simulink model "humanTestController"  (Simulink 9.1)
settings: Solver=FixedStepDiscrete  StartTime=0.0  StopTime=inf  FixedStep=Config.Ts  RelTol=1e-3  EnableMultiTasking=on
InitFcn:
  | initHumanController
values from neighbouring files (symbols this model uses):
  HUMAN_ON_GAZEBO = true    [initHumanController.m]
libraries: WBToolboxLibrary x17
settings Model: SuppressorTable=22 serialization::archive 11 0 6 0 0 0 1 0  Creator=yeshi  LastModifiedBy=yeshi
settings DataIOCC: SaveFormat=Dataset
settings DebuggingCC: UnderspecifiedInitializationDetection=Simplified  MergeDetectMultiDrivingBlocksExec=error
settings HardwareCC: ProdBitPerPointer=64  ProdBitPerSizeT=64  ProdBitPerPtrDiffT=64  ProdLargestAtomicFloat=Float  ProdIntDivRoundTo=Zero  ProdEndianess=LittleEndian  ProdWordSize=64  ProdHWDeviceType=Intel->x86-64 (Windows64)
settings ModelReferenceCC: PropagateSignalLabelsOutOfModel=on
settings GRTTargetCC: GeneratePreprocessorConditionals=Disable all  CombineOutputUpdateFcns=on  GRTInterface=off

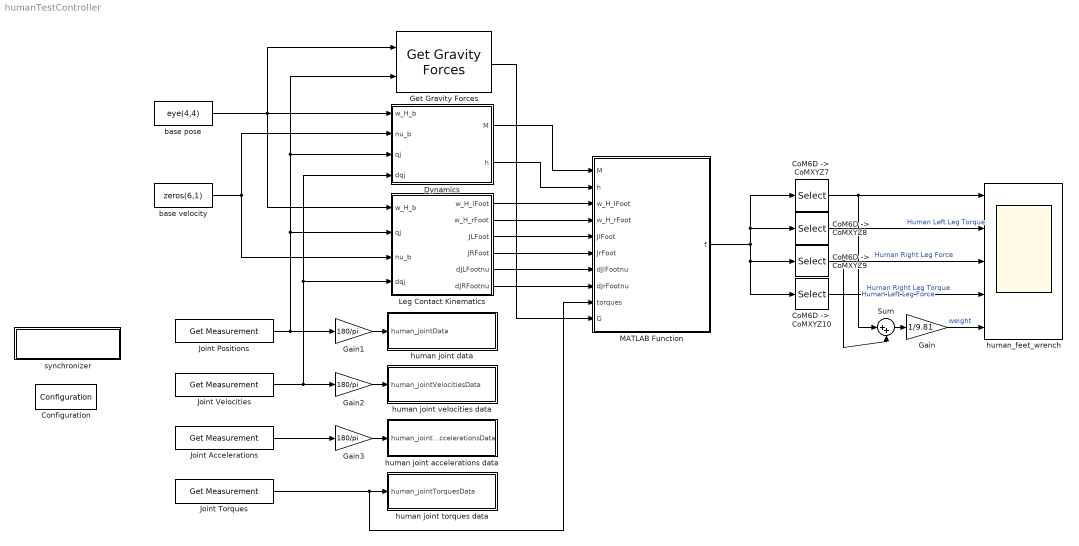
== system humanTestController ==
  "CoM6D ->  CoMXYZ10" : Selector  InputPortWidth=12  IndexOptions=Index vector (dialog)  Indices=[10 11 12]  OutputSizes=1
  "CoM6D ->  CoMXYZ7" : Selector  InputPortWidth=12  IndexOptions=Index vector (dialog)  Indices=[1 2 3]  OutputSizes=1
  "CoM6D ->  CoMXYZ8" : Selector  InputPortWidth=12  IndexOptions=Index vector (dialog)  Indices=[4 5 6]  OutputSizes=1
  "CoM6D ->  CoMXYZ9" : Selector  InputPortWidth=12  IndexOptions=Index vector (dialog)  Indices=[7 8 9]  OutputSizes=1
  Configuration : WBToolboxLibrary/Utilities/Configuration  ConfigSource=Workspace  ConfigObject='HUMAN.WBTConfigRobot'
      settings: SourceProductName=Whole Body Toolbox
  Dynamics : Subsystem
  Gain : Gain  Gain=1/9.81
  Gain1 : Gain  Gain=180/pi
  Gain2 : Gain  Gain=180/pi
  Gain3 : Gain  Gain=180/pi
  Get Gravity Forces : WBToolboxLibrary/wholeBodyModel/Dynamics/Get Gravity Forces
      settings: SourceProductName=Whole Body Toolbox
  Joint Accelerations : WBToolboxLibrary/wholeBodyStates/Get Measurement  measuredType=Joints Acceleration
      settings: SourceProductName=Whole Body Toolbox
  Joint Positions : WBToolboxLibrary/wholeBodyStates/Get Measurement  measuredType=Joints Position
      settings: SourceProductName=Whole Body Toolbox
  Joint Torques : WBToolboxLibrary/wholeBodyStates/Get Measurement  measuredType=Joints Torque
      settings: SourceProductName=Whole Body Toolbox
  Joint Velocities : WBToolboxLibrary/wholeBodyStates/Get Measurement  measuredType=Joints Velocity
      settings: SourceProductName=Whole Body Toolbox
  Leg Contact Kinematics : Subsystem
  MATLAB Function : MATLAB Function  TreatAsAtomicUnit=on
  Sum : Sum  Inputs=|++
  base pose : Constant  Value=eye(4,4)
  base velocity : Constant  Value=zeros(6,1)
  human joint accelerations data : Subsystem
  human joint data : Subsystem
  human joint torques data : Subsystem
  human joint velocities data : Subsystem
  human_feet_wrench : Scope  NumInputPorts=5
  synchronizer : Subsystem
      mask Display: disp('SYNCHRONIZER')
  wires:
  Joint Positions/1 -> Leg Contact Kinematics/2(qj), Dynamics/3(qj), Get Gravity Forces/2, Gain1/1
  Gain2/1 -> human joint velocities data/1(human_jointVelocitiesData)
  Gain3/1 -> human joint accelerations data/1(human_jointAccelerationsData)
  Joint Velocities/1 -> Leg Contact Kinematics/4(dqj), Dynamics/4(dqj), Gain2/1
  Joint Accelerations/1 -> Gain3/1
  Joint Torques/1 -> MATLAB Function/9(torques), human joint torques data/1(human_jointTorquesData)
  base pose/1 -> Dynamics/1(w_H_b), Get Gravity Forces/1, Leg Contact Kinematics/1(w_H_b)
  base velocity/1 -> Leg Contact Kinematics/3(nu_b), Dynamics/2(nu_b)
  Gain1/1 -> human joint data/1(human_jointData)
  Leg Contact Kinematics/1(w_H_lFoot) -> MATLAB Function/3(w_H_lFoot)
  Leg Contact Kinematics/2(w_H_rFoot) -> MATLAB Function/4(w_H_rFoot)
  Leg Contact Kinematics/3(JLFoot) -> MATLAB Function/5(JlFoot)
  Leg Contact Kinematics/4(JRFoot) -> MATLAB Function/6(JrFoot)
  Leg Contact Kinematics/5(dJLFootnu) -> MATLAB Function/7(dJlFootnu)
  Leg Contact Kinematics/6(dJRFootnu) -> MATLAB Function/8(dJrFootnu)
  Dynamics/2(h) -> MATLAB Function/2(h)
  Dynamics/1(M) -> MATLAB Function/1(M)
  "CoM6D ->  CoMXYZ8"/1 -> human_feet_wrench/2  "Human Left Leg Torque"
  MATLAB Function/1(f) -> "CoM6D ->  CoMXYZ10"/1, "CoM6D ->  CoMXYZ9"/1, "CoM6D ->  CoMXYZ8"/1, "CoM6D ->  CoMXYZ7"/1
  "CoM6D ->  CoMXYZ10"/1 -> human_feet_wrench/4  "Human Right Leg Torque"
  "CoM6D ->  CoMXYZ7"/1 -> Sum/1, human_feet_wrench/1  "Human Left Leg Force"
  "CoM6D ->  CoMXYZ9"/1 -> Sum/2, human_feet_wrench/3  "Human Right Leg Force"
  Get Gravity Forces/1 -> MATLAB Function/10(G)
  Sum/1 -> Gain/1
  Gain/1 -> human_feet_wrench/5  "weight"

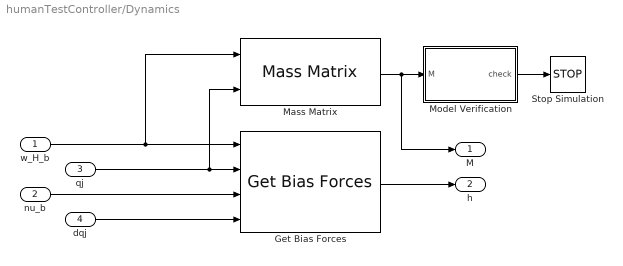
== system humanTestController/Dynamics ==
  w_H_b : Inport
  nu_b : Inport  Port=2
  qj : Inport  Port=3
  dqj : Inport  Port=4
  Get Bias Forces : WBToolboxLibrary/wholeBodyModel/Dynamics/Get Bias Forces
      settings: SourceProductName=Whole Body Toolbox
  Mass Matrix : WBToolboxLibrary/wholeBodyModel/Dynamics/Mass Matrix
      settings: SourceProductName=Whole Body Toolbox
  Model Verification : MATLAB Function  TreatAsAtomicUnit=on
  Stop Simulation : Stop
  M : Outport
  h : Outport  Port=2
  wires:
  dqj/1 -> Get Bias Forces/4
  w_H_b/1 -> Get Bias Forces/1, Mass Matrix/1
  qj/1 -> Get Bias Forces/2, Mass Matrix/2
  Mass Matrix/1 -> M/1, Model Verification/1(M)
  nu_b/1 -> Get Bias Forces/3
  Get Bias Forces/1 -> h/1
  Model Verification/1(check) -> Stop Simulation/1

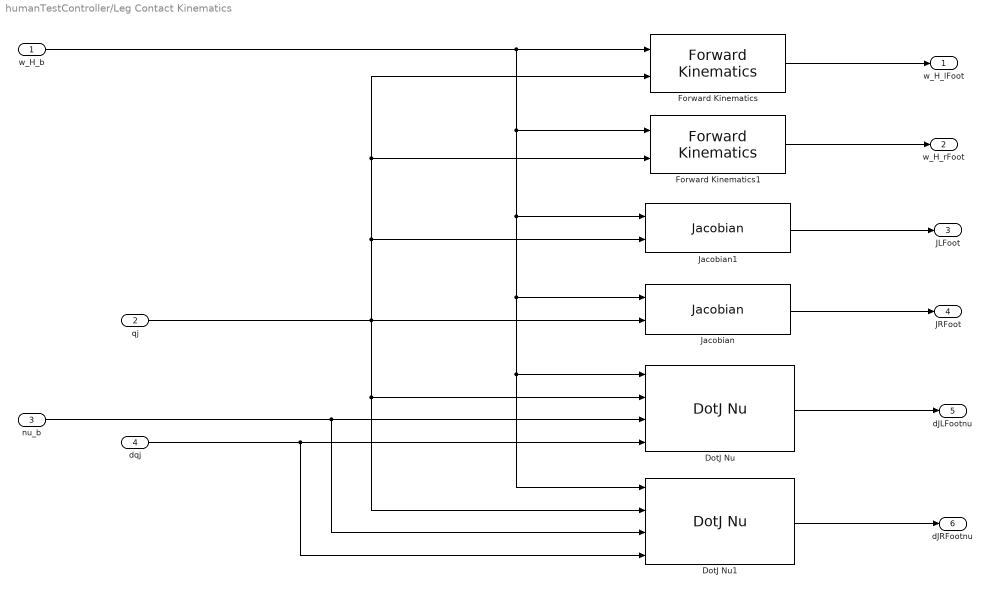
== system humanTestController/Leg Contact Kinematics ==
  w_H_b : Inport
  qj : Inport  Port=2
  nu_b : Inport  Port=3
  dqj : Inport  Port=4
  DotJ Nu : WBToolboxLibrary/wholeBodyModel/Jacobians/DotJ Nu  frameName=HUMAN_Frames.LEFT_FOOT
      settings: SourceProductName=Whole Body Toolbox
  DotJ Nu1 : WBToolboxLibrary/wholeBodyModel/Jacobians/DotJ Nu  frameName=HUMAN_Frames.RIGHT_FOOT
      settings: SourceProductName=Whole Body Toolbox
  Forward Kinematics : WBToolboxLibrary/wholeBodyModel/Kinematics/Forward Kinematics  frameName=HUMAN_Frames.LEFT_FOOT
      settings: SourceProductName=Whole Body Toolbox
  Forward Kinematics1 : WBToolboxLibrary/wholeBodyModel/Kinematics/Forward Kinematics  frameName=HUMAN_Frames.RIGHT_FOOT
      settings: SourceProductName=Whole Body Toolbox
  Jacobian : WBToolboxLibrary/wholeBodyModel/Jacobians/Jacobian  frameName=HUMAN_Frames.RIGHT_FOOT
      settings: SourceProductName=Whole Body Toolbox
  Jacobian1 : WBToolboxLibrary/wholeBodyModel/Jacobians/Jacobian  frameName=HUMAN_Frames.LEFT_FOOT
      settings: SourceProductName=Whole Body Toolbox
  w_H_lFoot : Outport
  w_H_rFoot : Outport  Port=2
  JLFoot : Outport  Port=3
  JRFoot : Outport  Port=4
  dJLFootnu : Outport  Port=5
  dJRFootnu : Outport  Port=6
  wires:
  DotJ Nu/1 -> dJLFootnu/1
  DotJ Nu1/1 -> dJRFootnu/1
  Jacobian/1 -> JRFoot/1
  Forward Kinematics1/1 -> w_H_rFoot/1
  nu_b/1 -> DotJ Nu1/3, DotJ Nu/3
  qj/1 -> Forward Kinematics/2, Forward Kinematics1/2, Jacobian1/2, Jacobian/2, DotJ Nu/2, DotJ Nu1/2
  w_H_b/1 -> Forward Kinematics1/1, Jacobian1/1, DotJ Nu/1, DotJ Nu1/1, Jacobian/1, Forward Kinematics/1
  dqj/1 -> DotJ Nu1/4, DotJ Nu/4
  Jacobian1/1 -> JLFoot/1
  Forward Kinematics/1 -> w_H_lFoot/1

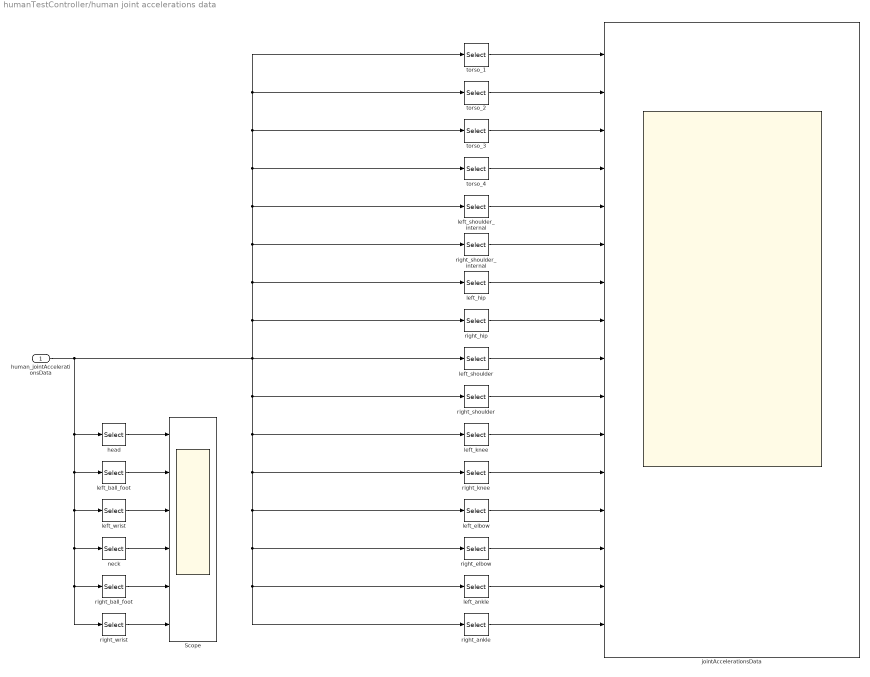
== system humanTestController/human joint accelerations data ==
  human_jointAccelerationsData : Inport
  Scope : Scope  NumInputPorts=6
  head : Selector  InputPortWidth=66  IndexOptions=Index vector (dialog)  Indices=[16 17 18]  OutputSizes=1
  jointAccelerationsData : Scope  NumInputPorts=16
  left_ankle : Selector  InputPortWidth=66  IndexOptions=Index vector (dialog)  Indices=[61 62 63]  OutputSizes=1
  left_ball_foot : Selector  InputPortWidth=66  IndexOptions=Index vector (dialog)  Indices=[64 65 66]  OutputSizes=1
  left_elbow : Selector  InputPortWidth=66  IndexOptions=Index vector (dialog)  Indices=[37 38 39]  OutputSizes=1
  left_hip : Selector  InputPortWidth=66  IndexOptions=Index vector (dialog)  Indices=[55 56 57]  OutputSizes=1
  left_knee : Selector  InputPortWidth=66  IndexOptions=Index vector (dialog)  Indices=[58 59 60]  OutputSizes=1
  left_shoulder : Selector  InputPortWidth=66  IndexOptions=Index vector (dialog)  Indices=[34 35 36]  OutputSizes=1
  left_shoulder_internal : Selector  InputPortWidth=66  IndexOptions=Index vector (dialog)  Indices=[31 32 33]  OutputSizes=1
  left_wrist : Selector  InputPortWidth=66  IndexOptions=Index vector (dialog)  Indices=[40 41 42]  OutputSizes=1
  neck : Selector  InputPortWidth=66  IndexOptions=Index vector (dialog)  Indices=[13 14 15]  OutputSizes=1
  right_ankle : Selector  InputPortWidth=66  IndexOptions=Index vector (dialog)  Indices=[49 50 51]  OutputSizes=1
  right_ball_foot : Selector  InputPortWidth=66  IndexOptions=Index vector (dialog)  Indices=[52 53 54]  OutputSizes=1
  right_elbow : Selector  InputPortWidth=66  IndexOptions=Index vector (dialog)  Indices=[25 26 27]  OutputSizes=1
  right_hip : Selector  InputPortWidth=66  IndexOptions=Index vector (dialog)  Indices=[43 44 45]  OutputSizes=1
  right_knee : Selector  InputPortWidth=66  IndexOptions=Index vector (dialog)  Indices=[46 47 48]  OutputSizes=1
  right_shoulder : Selector  InputPortWidth=66  IndexOptions=Index vector (dialog)  Indices=[22 23 24]  OutputSizes=1
  right_shoulder_internal : Selector  InputPortWidth=66  IndexOptions=Index vector (dialog)  Indices=[19 20 21]  OutputSizes=1
  right_wrist : Selector  InputPortWidth=66  IndexOptions=Index vector (dialog)  Indices=[28 29 30]  OutputSizes=1
  torso_1 : Selector  InputPortWidth=66  IndexOptions=Index vector (dialog)  Indices=[10 11 12]  OutputSizes=1
  torso_2 : Selector  InputPortWidth=66  IndexOptions=Index vector (dialog)  Indices=[7 8 9]  OutputSizes=1
  torso_3 : Selector  InputPortWidth=66  IndexOptions=Index vector (dialog)  Indices=[4 5 6]  OutputSizes=1
  torso_4 : Selector  InputPortWidth=66  IndexOptions=Index vector (dialog)  Indices=[1 2 3]  OutputSizes=1
  wires:
  torso_1/1 -> jointAccelerationsData/1
  torso_4/1 -> jointAccelerationsData/4
  torso_3/1 -> jointAccelerationsData/3
  torso_2/1 -> jointAccelerationsData/2
  right_shoulder_internal/1 -> jointAccelerationsData/6
  left_shoulder_internal/1 -> jointAccelerationsData/5
  left_hip/1 -> jointAccelerationsData/7
  right_hip/1 -> jointAccelerationsData/8
  left_shoulder/1 -> jointAccelerationsData/9
  right_shoulder/1 -> jointAccelerationsData/10
  left_knee/1 -> jointAccelerationsData/11
  right_knee/1 -> jointAccelerationsData/12
  left_elbow/1 -> jointAccelerationsData/13
  right_elbow/1 -> jointAccelerationsData/14
  left_ankle/1 -> jointAccelerationsData/15
  right_ankle/1 -> jointAccelerationsData/16
  human_jointAccelerationsData/1 -> head/1, left_ball_foot/1, left_wrist/1, neck/1, right_ball_foot/1, right_wrist/1, left_shoulder/1, right_hip/1, left_hip/1, right_shoulder_internal/1, torso_1/1, torso_2/1, torso_3/1, torso_4/1, left_shoulder_internal/1, right_shoulder/1, left_knee/1, right_knee/1, left_elbow/1, right_elbow/1, right_ankle/1, left_ankle/1
  head/1 -> Scope/1
  left_ball_foot/1 -> Scope/2
  left_wrist/1 -> Scope/3
  neck/1 -> Scope/4
  right_ball_foot/1 -> Scope/5
  right_wrist/1 -> Scope/6

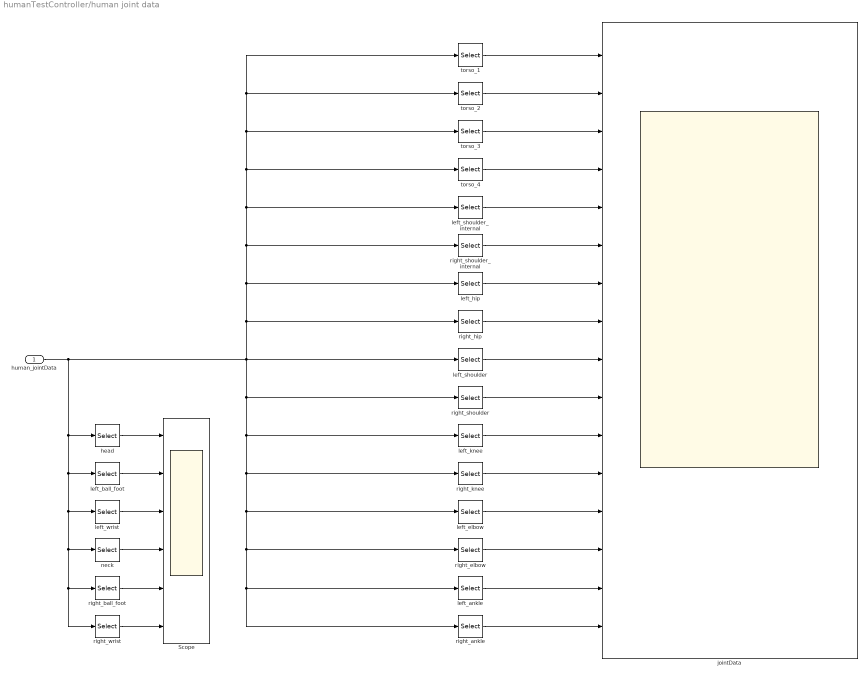
== system humanTestController/human joint data ==
  human_jointData : Inport
  Scope : Scope  NumInputPorts=6
  head : Selector  InputPortWidth=66  IndexOptions=Index vector (dialog)  Indices=[16 17 18]  OutputSizes=1
  jointData : Scope  NumInputPorts=16
  left_ankle : Selector  InputPortWidth=66  IndexOptions=Index vector (dialog)  Indices=[61 62 63]  OutputSizes=1
  left_ball_foot : Selector  InputPortWidth=66  IndexOptions=Index vector (dialog)  Indices=[64 65 66]  OutputSizes=1
  left_elbow : Selector  InputPortWidth=66  IndexOptions=Index vector (dialog)  Indices=[37 38 39]  OutputSizes=1
  left_hip : Selector  InputPortWidth=66  IndexOptions=Index vector (dialog)  Indices=[55 56 57]  OutputSizes=1
  left_knee : Selector  InputPortWidth=66  IndexOptions=Index vector (dialog)  Indices=[58 59 60]  OutputSizes=1
  left_shoulder : Selector  InputPortWidth=66  IndexOptions=Index vector (dialog)  Indices=[34 35 36]  OutputSizes=1
  left_shoulder_internal : Selector  InputPortWidth=66  IndexOptions=Index vector (dialog)  Indices=[31 32 33]  OutputSizes=1
  left_wrist : Selector  InputPortWidth=66  IndexOptions=Index vector (dialog)  Indices=[40 41 42]  OutputSizes=1
  neck : Selector  InputPortWidth=66  IndexOptions=Index vector (dialog)  Indices=[13 14 15]  OutputSizes=1
  right_ankle : Selector  InputPortWidth=66  IndexOptions=Index vector (dialog)  Indices=[49 50 51]  OutputSizes=1
  right_ball_foot : Selector  InputPortWidth=66  IndexOptions=Index vector (dialog)  Indices=[52 53 54]  OutputSizes=1
  right_elbow : Selector  InputPortWidth=66  IndexOptions=Index vector (dialog)  Indices=[25 26 27]  OutputSizes=1
  right_hip : Selector  InputPortWidth=66  IndexOptions=Index vector (dialog)  Indices=[43 44 45]  OutputSizes=1
  right_knee : Selector  InputPortWidth=66  IndexOptions=Index vector (dialog)  Indices=[46 47 48]  OutputSizes=1
  right_shoulder : Selector  InputPortWidth=66  IndexOptions=Index vector (dialog)  Indices=[22 23 24]  OutputSizes=1
  right_shoulder_internal : Selector  InputPortWidth=66  IndexOptions=Index vector (dialog)  Indices=[19 20 21]  OutputSizes=1
  right_wrist : Selector  InputPortWidth=66  IndexOptions=Index vector (dialog)  Indices=[28 29 30]  OutputSizes=1
  torso_1 : Selector  InputPortWidth=66  IndexOptions=Index vector (dialog)  Indices=[10 11 12]  OutputSizes=1
  torso_2 : Selector  InputPortWidth=66  IndexOptions=Index vector (dialog)  Indices=[7 8 9]  OutputSizes=1
  torso_3 : Selector  InputPortWidth=66  IndexOptions=Index vector (dialog)  Indices=[4 5 6]  OutputSizes=1
  torso_4 : Selector  InputPortWidth=66  IndexOptions=Index vector (dialog)  Indices=[1 2 3]  OutputSizes=1
  wires:
  torso_1/1 -> jointData/1
  torso_4/1 -> jointData/4
  torso_3/1 -> jointData/3
  torso_2/1 -> jointData/2
  right_shoulder_internal/1 -> jointData/6
  left_shoulder_internal/1 -> jointData/5
  left_hip/1 -> jointData/7
  right_hip/1 -> jointData/8
  left_shoulder/1 -> jointData/9
  right_shoulder/1 -> jointData/10
  left_knee/1 -> jointData/11
  right_knee/1 -> jointData/12
  left_elbow/1 -> jointData/13
  right_elbow/1 -> jointData/14
  left_ankle/1 -> jointData/15
  right_ankle/1 -> jointData/16
  human_jointData/1 -> head/1, left_ball_foot/1, left_wrist/1, neck/1, right_ball_foot/1, right_wrist/1, left_shoulder/1, right_hip/1, left_hip/1, right_shoulder_internal/1, torso_1/1, torso_2/1, torso_3/1, torso_4/1, left_shoulder_internal/1, right_shoulder/1, left_knee/1, right_knee/1, left_elbow/1, right_elbow/1, right_ankle/1, left_ankle/1
  head/1 -> Scope/1
  left_ball_foot/1 -> Scope/2
  left_wrist/1 -> Scope/3
  neck/1 -> Scope/4
  right_ball_foot/1 -> Scope/5
  right_wrist/1 -> Scope/6

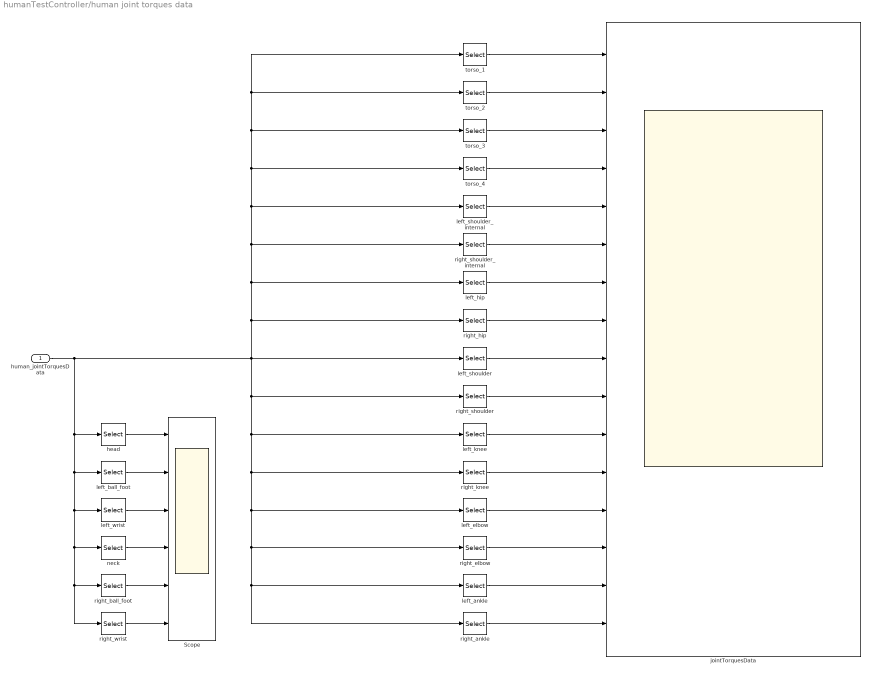
== system humanTestController/human joint torques data ==
  human_jointTorquesData : Inport
  Scope : Scope  NumInputPorts=6
  head : Selector  InputPortWidth=66  IndexOptions=Index vector (dialog)  Indices=[16 17 18]  OutputSizes=1
  jointTorquesData : Scope  NumInputPorts=16
  left_ankle : Selector  InputPortWidth=66  IndexOptions=Index vector (dialog)  Indices=[61 62 63]  OutputSizes=1
  left_ball_foot : Selector  InputPortWidth=66  IndexOptions=Index vector (dialog)  Indices=[64 65 66]  OutputSizes=1
  left_elbow : Selector  InputPortWidth=66  IndexOptions=Index vector (dialog)  Indices=[37 38 39]  OutputSizes=1
  left_hip : Selector  InputPortWidth=66  IndexOptions=Index vector (dialog)  Indices=[55 56 57]  OutputSizes=1
  left_knee : Selector  InputPortWidth=66  IndexOptions=Index vector (dialog)  Indices=[58 59 60]  OutputSizes=1
  left_shoulder : Selector  InputPortWidth=66  IndexOptions=Index vector (dialog)  Indices=[34 35 36]  OutputSizes=1
  left_shoulder_internal : Selector  InputPortWidth=66  IndexOptions=Index vector (dialog)  Indices=[31 32 33]  OutputSizes=1
  left_wrist : Selector  InputPortWidth=66  IndexOptions=Index vector (dialog)  Indices=[40 41 42]  OutputSizes=1
  neck : Selector  InputPortWidth=66  IndexOptions=Index vector (dialog)  Indices=[13 14 15]  OutputSizes=1
  right_ankle : Selector  InputPortWidth=66  IndexOptions=Index vector (dialog)  Indices=[49 50 51]  OutputSizes=1
  right_ball_foot : Selector  InputPortWidth=66  IndexOptions=Index vector (dialog)  Indices=[52 53 54]  OutputSizes=1
  right_elbow : Selector  InputPortWidth=66  IndexOptions=Index vector (dialog)  Indices=[25 26 27]  OutputSizes=1
  right_hip : Selector  InputPortWidth=66  IndexOptions=Index vector (dialog)  Indices=[43 44 45]  OutputSizes=1
  right_knee : Selector  InputPortWidth=66  IndexOptions=Index vector (dialog)  Indices=[46 47 48]  OutputSizes=1
  right_shoulder : Selector  InputPortWidth=66  IndexOptions=Index vector (dialog)  Indices=[22 23 24]  OutputSizes=1
  right_shoulder_internal : Selector  InputPortWidth=66  IndexOptions=Index vector (dialog)  Indices=[19 20 21]  OutputSizes=1
  right_wrist : Selector  InputPortWidth=66  IndexOptions=Index vector (dialog)  Indices=[28 29 30]  OutputSizes=1
  torso_1 : Selector  InputPortWidth=66  IndexOptions=Index vector (dialog)  Indices=[10 11 12]  OutputSizes=1
  torso_2 : Selector  InputPortWidth=66  IndexOptions=Index vector (dialog)  Indices=[7 8 9]  OutputSizes=1
  torso_3 : Selector  InputPortWidth=66  IndexOptions=Index vector (dialog)  Indices=[4 5 6]  OutputSizes=1
  torso_4 : Selector  InputPortWidth=66  IndexOptions=Index vector (dialog)  Indices=[1 2 3]  OutputSizes=1
  wires:
  torso_1/1 -> jointTorquesData/1
  torso_4/1 -> jointTorquesData/4
  torso_3/1 -> jointTorquesData/3
  torso_2/1 -> jointTorquesData/2
  right_shoulder_internal/1 -> jointTorquesData/6
  left_shoulder_internal/1 -> jointTorquesData/5
  left_hip/1 -> jointTorquesData/7
  right_hip/1 -> jointTorquesData/8
  left_shoulder/1 -> jointTorquesData/9
  right_shoulder/1 -> jointTorquesData/10
  left_knee/1 -> jointTorquesData/11
  right_knee/1 -> jointTorquesData/12
  left_elbow/1 -> jointTorquesData/13
  right_elbow/1 -> jointTorquesData/14
  left_ankle/1 -> jointTorquesData/15
  right_ankle/1 -> jointTorquesData/16
  human_jointTorquesData/1 -> head/1, left_ball_foot/1, left_wrist/1, neck/1, right_ball_foot/1, right_wrist/1, left_shoulder/1, right_hip/1, left_hip/1, right_shoulder_internal/1, torso_1/1, torso_2/1, torso_3/1, torso_4/1, left_shoulder_internal/1, right_shoulder/1, left_knee/1, right_knee/1, left_elbow/1, right_elbow/1, right_ankle/1, left_ankle/1
  head/1 -> Scope/1
  left_ball_foot/1 -> Scope/2
  left_wrist/1 -> Scope/3
  neck/1 -> Scope/4
  right_ball_foot/1 -> Scope/5
  right_wrist/1 -> Scope/6

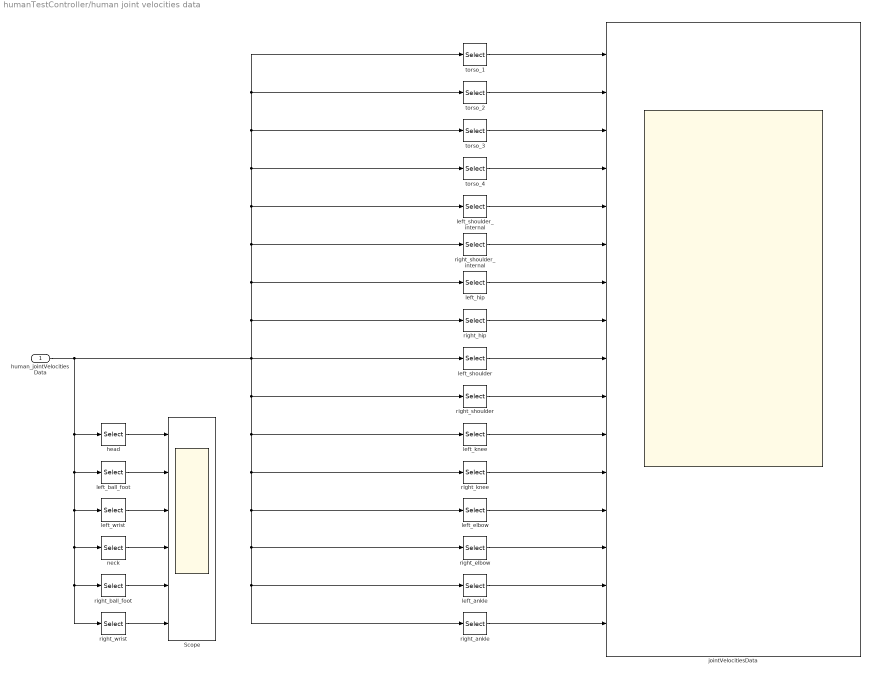
== system humanTestController/human joint velocities data ==
  human_jointVelocitiesData : Inport
  Scope : Scope  NumInputPorts=6
  head : Selector  InputPortWidth=66  IndexOptions=Index vector (dialog)  Indices=[16 17 18]  OutputSizes=1
  jointVelocitiesData : Scope  NumInputPorts=16
  left_ankle : Selector  InputPortWidth=66  IndexOptions=Index vector (dialog)  Indices=[61 62 63]  OutputSizes=1
  left_ball_foot : Selector  InputPortWidth=66  IndexOptions=Index vector (dialog)  Indices=[64 65 66]  OutputSizes=1
  left_elbow : Selector  InputPortWidth=66  IndexOptions=Index vector (dialog)  Indices=[37 38 39]  OutputSizes=1
  left_hip : Selector  InputPortWidth=66  IndexOptions=Index vector (dialog)  Indices=[55 56 57]  OutputSizes=1
  left_knee : Selector  InputPortWidth=66  IndexOptions=Index vector (dialog)  Indices=[58 59 60]  OutputSizes=1
  left_shoulder : Selector  InputPortWidth=66  IndexOptions=Index vector (dialog)  Indices=[34 35 36]  OutputSizes=1
  left_shoulder_internal : Selector  InputPortWidth=66  IndexOptions=Index vector (dialog)  Indices=[31 32 33]  OutputSizes=1
  left_wrist : Selector  InputPortWidth=66  IndexOptions=Index vector (dialog)  Indices=[40 41 42]  OutputSizes=1
  neck : Selector  InputPortWidth=66  IndexOptions=Index vector (dialog)  Indices=[13 14 15]  OutputSizes=1
  right_ankle : Selector  InputPortWidth=66  IndexOptions=Index vector (dialog)  Indices=[49 50 51]  OutputSizes=1
  right_ball_foot : Selector  InputPortWidth=66  IndexOptions=Index vector (dialog)  Indices=[52 53 54]  OutputSizes=1
  right_elbow : Selector  InputPortWidth=66  IndexOptions=Index vector (dialog)  Indices=[25 26 27]  OutputSizes=1
  right_hip : Selector  InputPortWidth=66  IndexOptions=Index vector (dialog)  Indices=[43 44 45]  OutputSizes=1
  right_knee : Selector  InputPortWidth=66  IndexOptions=Index vector (dialog)  Indices=[46 47 48]  OutputSizes=1
  right_shoulder : Selector  InputPortWidth=66  IndexOptions=Index vector (dialog)  Indices=[22 23 24]  OutputSizes=1
  right_shoulder_internal : Selector  InputPortWidth=66  IndexOptions=Index vector (dialog)  Indices=[19 20 21]  OutputSizes=1
  right_wrist : Selector  InputPortWidth=66  IndexOptions=Index vector (dialog)  Indices=[28 29 30]  OutputSizes=1
  torso_1 : Selector  InputPortWidth=66  IndexOptions=Index vector (dialog)  Indices=[10 11 12]  OutputSizes=1
  torso_2 : Selector  InputPortWidth=66  IndexOptions=Index vector (dialog)  Indices=[7 8 9]  OutputSizes=1
  torso_3 : Selector  InputPortWidth=66  IndexOptions=Index vector (dialog)  Indices=[4 5 6]  OutputSizes=1
  torso_4 : Selector  InputPortWidth=66  IndexOptions=Index vector (dialog)  Indices=[1 2 3]  OutputSizes=1
  wires:
  torso_1/1 -> jointVelocitiesData/1
  torso_4/1 -> jointVelocitiesData/4
  torso_3/1 -> jointVelocitiesData/3
  torso_2/1 -> jointVelocitiesData/2
  right_shoulder_internal/1 -> jointVelocitiesData/6
  left_shoulder_internal/1 -> jointVelocitiesData/5
  left_hip/1 -> jointVelocitiesData/7
  right_hip/1 -> jointVelocitiesData/8
  left_shoulder/1 -> jointVelocitiesData/9
  right_shoulder/1 -> jointVelocitiesData/10
  left_knee/1 -> jointVelocitiesData/11
  right_knee/1 -> jointVelocitiesData/12
  left_elbow/1 -> jointVelocitiesData/13
  right_elbow/1 -> jointVelocitiesData/14
  left_ankle/1 -> jointVelocitiesData/15
  right_ankle/1 -> jointVelocitiesData/16
  human_jointVelocitiesData/1 -> head/1, left_ball_foot/1, left_wrist/1, neck/1, right_ball_foot/1, right_wrist/1, left_shoulder/1, right_hip/1, left_hip/1, right_shoulder_internal/1, torso_1/1, torso_2/1, torso_3/1, torso_4/1, left_shoulder_internal/1, right_shoulder/1, left_knee/1, right_knee/1, left_elbow/1, right_elbow/1, right_ankle/1, left_ankle/1
  head/1 -> Scope/1
  left_ball_foot/1 -> Scope/2
  left_wrist/1 -> Scope/3
  neck/1 -> Scope/4
  right_ball_foot/1 -> Scope/5
  right_wrist/1 -> Scope/6

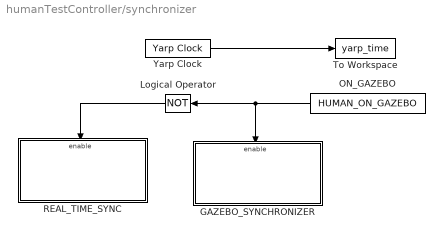
== system humanTestController/synchronizer ==
  GAZEBO_SYNCHRONIZER : Subsystem
  Logical Operator : Logic  Operator=NOT  AllPortsSameDT=off  OutDataTypeStr=boolean
  "ON_GAZEBO " : Constant  Value=HUMAN_ON_GAZEBO
  REAL_TIME_SYNC : Subsystem
  To Workspace : ToWorkspace  VariableName=yarp_time  SaveFormat=Structure With Time  SampleTime=-1
  Yarp Clock : WBToolboxLibrary/Utilities/Yarp Clock
      settings: SourceProductName=Whole Body Toolbox
  wires:
  Logical Operator/1 -> REAL_TIME_SYNC/Enable
  "ON_GAZEBO "/1 -> GAZEBO_SYNCHRONIZER/Enable, Logical Operator/1
  Yarp Clock/1 -> To Workspace/1

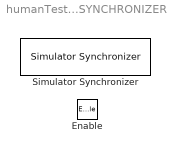
== system humanTestController/synchronizer/GAZEBO_SYNCHRONIZER ==
  Enable : EnablePort
  Simulator Synchronizer : WBToolboxLibrary/Utilities/Simulator Synchronizer  period=Config.Ts  serverPortName='/clock/rpc'  clientPortName='/WBT_synchronizer/rpc:o'
      settings: SourceProductName=Whole Body Toolbox

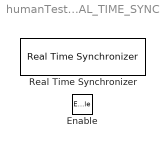
== system humanTestController/synchronizer/REAL_TIME_SYNC ==
  Enable : EnablePort
  Real Time Synchronizer : WBToolboxLibrary/Utilities/Real Time Synchronizer  period=Config.Ts
      settings: SourceProductName=Whole Body Toolbox

== matlab function MATLAB Function ==
  data: M input double; f output double; h input double; w_H_lFoot input double; w_H_rFoot input double; JlFoot input double; JrFoot input double; dJlFootnu input double; dJrFootnu input double; torques input double; G input double
function f = computeContactWrench(M,h, w_H_lFoot, w_H_rFoot, JlFoot, JrFoot, dJlFootnu, dJrFootnu, torques, G)

    DoF = 66;

    % Mass of the human
    m              = M(1,1);
    
    gravAcc        = 9.81;
    
    St             = [zeros(6,DoF);
                      eye(DoF,DoF)];
                  
    gravityWrench  = [zeros(2,1);
                     -m*gravAcc;
                      zeros(3,1)];
                  
    % Time varying contact jacobian
    Jc              = [JlFoot;      
                       JrFoot];
                   
    % Time varying dot(J)*nu
    Jc_nuDot        = [dJlFootnu;      
                       dJrFootnu];
                   
    JcMinv          = Jc/(M+blkdiag(zeros(6),0.1*eye(DoF)));
    JcMinvJct       = JcMinv*transpose(Jc);
    
%     f = - (eye(12)/(JcMinvJct+0.000001*eye(12)))*(JcMinv * (St*torques-h) + Jc_nuDot); 


    f = (eye(12)/(Jc*transpose(Jc) + 0.001*eye(12)))*Jc*(G-St*torques);

end

== matlab function Dynamics/Model Verification ==
  data: M input double; check output double
function check  = verifyModel(M)

    check = 0;
    val = 0;
    %% Mass matrix is symmetric and positive definite
    [s,v,d] = svd(M);
    
    if(min(v(:)) < 0)
        check = 1;
        fprintf('Human model verification failed \n');
    end
    
end
